simulink model "sampleModel1715"  (R2023a)
settings: Solver=VariableStepAuto  StartTime=0.0  StopTime=10.0  RelTol=1e-3
libraries: hdlsllib x7
settings Model: Creator=user1  LastModifiedBy=user1

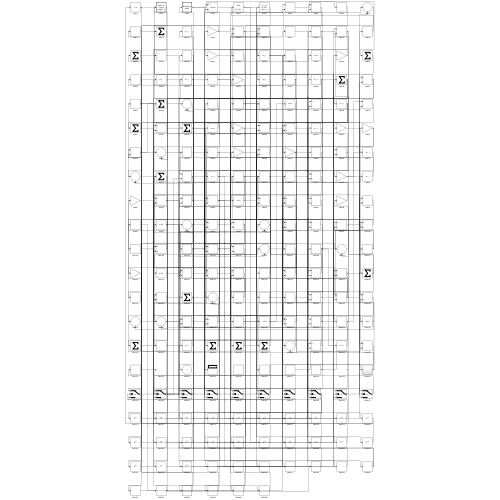
[thumbnail: Simulink's stored preview of the top-level diagram]
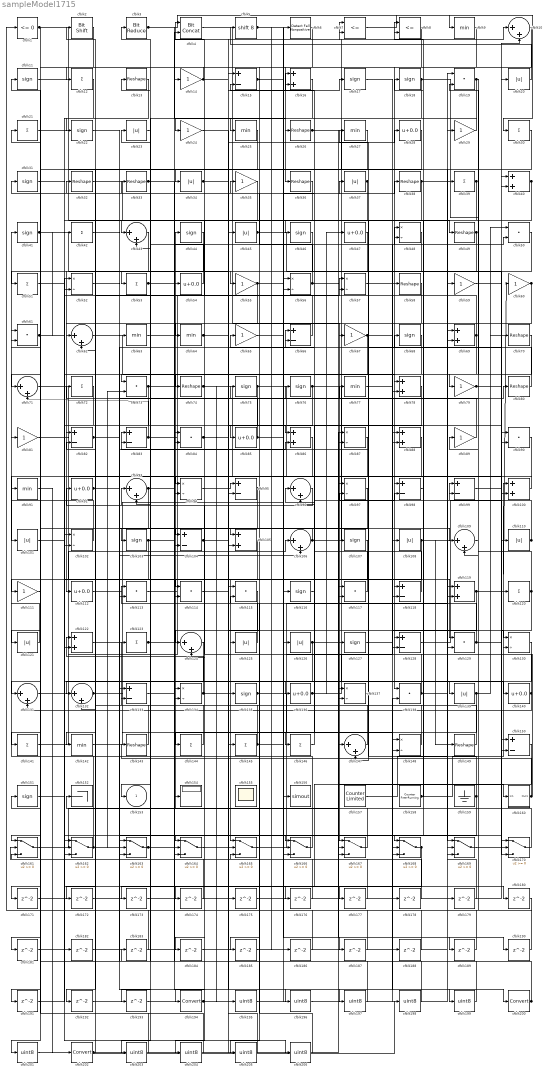
== system sampleModel1715 ==
  cfblk1 : hdlsllib/Logic and Bit Operations/Compare To Zero  relop=<=  OutDataTypeStr=boolean
  cfblk{10,43,62,71,93,96,106,109,124,131..132,147} (12 alike) : Sum  Inputs=|++
  cfblk{16,40,69,78,86,88,100,105,119,122} (10 alike) : Sum
  cfblk{20,23,34,37,45,101,108,110,121,125..126,139} (12 alike) : Abs  SaturateOnIntegerOverflow=off
  cfblk{48,52,56..57,87,94,97,102,130,134,137,148} (12 alike) : Product  Inputs=*/  RndMeth=Zero  SaturateOnIntegerOverflow=on
  cfblk{11,17..18,22,31,41,44,46,68,75..76,103,107,116,127,135,151} (17 alike) : Signum
  cfblk{15,66,82..83,95,98..99,104,118,128,133,150} (12 alike) : Sum  Inputs=+-
  cfblk{14,24,29,35,55,59..60,65,67,79,81,89,111} (13 alike) : Gain
  cfblk{28,47,54,85,92,112,136,140} (8 alike) : Bias  Bias=0.0  SaturateOnIntegerOverflow=off
  cfblk{19,50,61,73,84,90,113..115,117,129,138} (12 alike) : DotProduct  OutDataTypeStr=Inherit: Inherit via internal rule
  cfblk{12,21,30,39,42,51,53,72,120,123,141,144..146} (14 alike) : Sum  Inputs=+
  cfblk{13,26,32..33,36,38,49,58,70,74,80,143,149} (13 alike) : Reshape
  cfblk{9,25,27,63..64,77,91,142} (8 alike) : MinMax
  cfblk152 : Terminator
  cfblk154 : Display
  cfblk155 : Scope
      settings: Floating=on
  cfblk156 : ToWorkspace  VariableName=simout  SaveFormat=Timeseries  SampleTime=-1
  cfblk157 : hdlsllib/Sources/Counter Limited  uplimit=7  tsamp=-1
  cfblk158 : hdlsllib/Sources/Counter Free-Running  NumBits=16  tsamp=-1
  cfblk159 : Ground
  cfblk160 : Subsystem
      settings: LibrarySourceBlock=|
      | hdlsllib/Ports &
      | Subsystems/Subsystem
  cfblk{161..170} (10 alike) : Switch  SaturateOnIntegerOverflow=off  InputSameDT=off
  cfblk{171..193} (23 alike) : Delay  SampleTime=1
  cfblk194 : DataTypeConversion  SaturateOnIntegerOverflow=off  RndMeth=Floor
  cfblk{195..199,201,203..206} (10 alike) : DataTypeConversion  OutDataTypeStr=uint8  SaturateOnIntegerOverflow=off  RndMeth=Floor
  cfblk2 : hdlsllib/Logic and Bit Operations/Bit Shift  mode=Shift Left Logical  N=0
  cfblk200 : DataTypeConversion  SaturateOnIntegerOverflow=off  RndMeth=Floor
  cfblk202 : DataTypeConversion  SaturateOnIntegerOverflow=off  RndMeth=Floor
  cfblk3 : hdlsllib/Logic and Bit Operations/Bit Reduce  mode=AND
  cfblk4 : hdlsllib/Logic and Bit Operations/Bit Concat  numInputs=2
  cfblk5 : ArithShift  BitShiftNumber=8
  cfblk6 : hdlsllib/Logic and Bit Operations/Detect Fall Nonpositive  vinit=0  OutDataTypeStr=boolean
  cfblk7 : RelationalOperator  Operator=<=  OutDataTypeStr=boolean  InputSameDT=off
  cfblk8 : RelationalOperator  Operator=<=  OutDataTypeStr=boolean  InputSameDT=off
  cfblk153 : Outport  VectorParamsAs1DForOutWhenUnconnected=off
  wires:
  cfblk166/1 -> cfblk41/1
  cfblk27/1 -> cfblk34/1
  cfblk11/1 -> cfblk49/1
  cfblk18/1 -> cfblk53/1, cfblk88/2
  cfblk131/1 -> cfblk106/1
  cfblk116/1 -> cfblk65/1
  cfblk127/1 -> cfblk200/1
  cfblk149/1 -> cfblk96/1
  cfblk76/1 -> cfblk139/1, cfblk85/1
  cfblk5/1 -> cfblk186/1, cfblk187/1
  cfblk159/1 -> cfblk83/1, cfblk162/3
  cfblk82/1 -> cfblk66/1, cfblk109/1
  cfblk28/1 -> cfblk141/1
  cfblk143/1 -> cfblk32/1
  cfblk168/1 -> cfblk173/1, cfblk174/1
  cfblk110/1 -> cfblk99/1, cfblk75/1
  cfblk48/1 -> cfblk138/1
  cfblk50/1 -> cfblk112/1
  cfblk162/1 -> cfblk61/1, cfblk84/2, cfblk76/1, cfblk73/2, cfblk166/1, cfblk166/2
  cfblk121/1 -> cfblk81/1
  cfblk55/1 -> cfblk116/1, cfblk95/2
  cfblk4/1 -> cfblk167/1
  cfblk119/1 -> cfblk60/1, cfblk128/2
  cfblk106/1 -> cfblk10/1, cfblk105/1
  cfblk87/1 -> cfblk194/1
  cfblk138/1 -> cfblk59/1, cfblk92/1
  cfblk98/1 -> cfblk168/1
  cfblk167/1 -> cfblk44/1
  cfblk9/1 -> cfblk36/1
  cfblk75/1 -> cfblk168/2, cfblk170/1, cfblk132/2
  cfblk134/1 -> cfblk122/1, cfblk16/2
  cfblk86/1 -> cfblk101/1
  cfblk54/1 -> cfblk23/1
  cfblk165/1 -> cfblk29/1
  cfblk170/1 -> cfblk152/1
  cfblk26/1 -> cfblk88/1, cfblk160/1(In1), cfblk190/1
  cfblk47/1 -> cfblk51/1
  cfblk147/1 -> cfblk54/1
  cfblk141/1 -> cfblk6/1
  cfblk146/1 -> cfblk66/2
  cfblk49/1 -> cfblk104/1, cfblk117/2, cfblk104/2
  cfblk10/1 -> cfblk118/1
  cfblk104/1 -> cfblk15/1, cfblk129/2
  cfblk73/1 -> cfblk154/1, cfblk142/1
  cfblk38/1 -> cfblk64/1, cfblk78/2, cfblk130/1
  cfblk1/1 -> cfblk69/2, cfblk131/1
  cfblk88/1 -> cfblk121/1
  cfblk16/1 -> cfblk43/1
  cfblk107/1 -> cfblk165/1
  cfblk19/1 -> cfblk25/1, cfblk79/1
  cfblk83/1 -> cfblk40/1, cfblk71/2
  cfblk29/1 -> cfblk24/1
  cfblk129/1 -> cfblk20/1, cfblk27/1, cfblk13/1
  cfblk32/1 -> cfblk135/1
  cfblk161/1 -> cfblk107/1
  cfblk60/1 -> cfblk67/1, cfblk147/2
  cfblk15/1 -> cfblk126/1, cfblk185/1
  cfblk52/1 -> cfblk163/1
  cfblk2/1 -> cfblk71/1
  cfblk102/1 -> cfblk21/1
  cfblk128/1 -> cfblk10/2
  cfblk118/1 -> cfblk31/1
  cfblk80/1 -> cfblk57/1
  cfblk78/1 -> cfblk146/1
  cfblk126/1 -> cfblk96/2, cfblk98/2, cfblk164/2
  cfblk122/1 -> cfblk37/1
  cfblk158/1 -> cfblk100/1, cfblk18/1
  cfblk135/1 -> cfblk108/1, cfblk168/3
  cfblk93/1 -> cfblk14/1, cfblk113/2
  cfblk84/1 -> cfblk48/2, cfblk195/1, cfblk199/1
  cfblk13/1 -> cfblk122/2
  cfblk144/1 -> cfblk43/2
  cfblk151/1 -> cfblk57/2
  cfblk62/1 -> cfblk74/1
  cfblk3/1 -> cfblk30/1, cfblk26/1
  cfblk59/1 -> cfblk150/1
  cfblk109/1 -> cfblk19/2
  cfblk163/1 -> cfblk83/2, cfblk86/2
  cfblk113/1 -> cfblk68/1
  cfblk132/1 -> cfblk38/1, cfblk156/1
  cfblk81/1 -> cfblk129/1
  cfblk8/1 -> cfblk55/1
  cfblk21/1 -> cfblk169/1
  cfblk85/1 -> cfblk33/1, cfblk7/2
  cfblk99/1 -> cfblk90/1
  cfblk25/1 -> cfblk62/1
  cfblk43/1 -> cfblk111/1
  cfblk105/1 -> cfblk144/1
  cfblk64/1 -> cfblk86/1, cfblk184/1
  cfblk7/1 -> cfblk9/1
  cfblk42/1 -> cfblk63/1
  cfblk140/1 -> cfblk97/2, cfblk131/2
  cfblk31/1 -> cfblk114/1
  cfblk12/1 -> cfblk22/1
  cfblk164/1 -> cfblk28/1
  cfblk67/1 -> cfblk134/2, cfblk50/2
  cfblk91/1 -> cfblk202/1
  cfblk61/1 -> cfblk140/1, cfblk42/1
  cfblk97/1 -> cfblk161/1
  cfblk103/1 -> cfblk8/2, cfblk48/1, cfblk192/1
  cfblk33/1 -> cfblk103/1, cfblk105/2
  cfblk69/1 -> cfblk4/1, cfblk102/2
  cfblk71/1 -> cfblk100/2
  cfblk89/1 -> cfblk8/1
  cfblk94/1 -> cfblk95/1
  cfblk44/1 -> cfblk73/1
  cfblk123/1 -> cfblk4/2, cfblk193/1
  cfblk157/1 -> cfblk39/1
  cfblk45/1 -> cfblk110/1, cfblk170/2
  cfblk41/1 -> cfblk145/1, cfblk206/1
  cfblk108/1 -> cfblk149/1, cfblk40/2, cfblk191/1
  cfblk14/1 -> cfblk7/1, cfblk12/1
  cfblk46/1 -> cfblk93/2
  cfblk30/1 -> cfblk119/2
  cfblk112/1 -> cfblk56/2
  cfblk56/1 -> cfblk35/1, cfblk118/2, cfblk16/1
  cfblk74/1 -> cfblk98/1, cfblk175/1
  cfblk63/1 -> cfblk114/2
  cfblk100/1 -> cfblk94/1
  cfblk34/1 -> cfblk17/1, cfblk137/1
  cfblk142/1 -> cfblk147/1
  cfblk40/1 -> cfblk125/1, cfblk82/1
  cfblk95/1 -> cfblk124/2, cfblk171/1
  cfblk136/1 -> cfblk58/1, cfblk47/1
  cfblk96/1 -> cfblk94/2
  cfblk79/1 -> cfblk150/2, cfblk70/1
  cfblk90/1 -> cfblk148/2
  cfblk70/1 -> cfblk124/1
  cfblk137/1 -> cfblk77/1
  cfblk58/1 -> cfblk62/2
  cfblk169/1 -> cfblk120/1
  cfblk160/1(Out1) -> cfblk143/1, cfblk130/2
  cfblk120/1 -> cfblk72/1, cfblk89/1, cfblk170/3
  cfblk148/1 -> cfblk3/1
  cfblk23/1 -> cfblk153/1
  cfblk35/1 -> cfblk132/1
  cfblk20/1 -> cfblk5/1
  cfblk125/1 -> cfblk113/1
  cfblk53/1 -> cfblk78/1, cfblk137/2
  cfblk92/1 -> cfblk106/2, cfblk136/1
  cfblk72/1 -> cfblk162/2
  cfblk39/1 -> cfblk117/1, cfblk163/3, cfblk128/1
  cfblk66/1 -> cfblk2/1
  cfblk139/1 -> cfblk164/1, cfblk50/1, cfblk109/2
  cfblk65/1 -> cfblk167/2
  cfblk37/1 -> cfblk52/2, cfblk164/3
  cfblk24/1 -> cfblk46/1
  cfblk117/1 -> cfblk15/2
  cfblk68/1 -> cfblk167/3
  cfblk145/1 -> cfblk123/1, cfblk80/1
  cfblk171/1 -> cfblk163/2
  cfblk124/1 -> cfblk172/1
  cfblk172/1 -> cfblk148/1
  cfblk173/1 -> cfblk19/1
  cfblk174/1 -> cfblk161/2
  cfblk175/1 -> cfblk90/2
  cfblk150/1 -> cfblk176/1
  cfblk176/1 -> cfblk52/1
  cfblk101/1 -> cfblk177/1
  cfblk177/1 -> cfblk134/1
  cfblk57/1 -> cfblk178/1
  cfblk178/1 -> cfblk165/2
  cfblk179/1 -> cfblk69/1
  cfblk114/1 -> cfblk180/1
  cfblk180/1 -> cfblk1/1
  cfblk111/1 -> cfblk181/1
  cfblk181/1 -> cfblk119/1
  cfblk51/1 -> cfblk182/1
  cfblk182/1 -> cfblk169/3
  cfblk183/1 -> cfblk61/2
  cfblk184/1 -> cfblk56/1
  cfblk185/1 -> cfblk165/3
  cfblk186/1 -> cfblk93/1
  cfblk187/1 -> cfblk161/3
  cfblk17/1 -> cfblk188/1
  cfblk188/1 -> cfblk97/1
  cfblk77/1 -> cfblk189/1
  cfblk189/1 -> cfblk162/1
  cfblk190/1 -> cfblk99/2
  cfblk191/1 -> cfblk102/1
  cfblk192/1 -> cfblk169/2
  cfblk193/1 -> cfblk166/3
  cfblk194/1 -> cfblk179/1, cfblk138/2
  cfblk195/1 -> cfblk87/1
  cfblk22/1 -> cfblk196/1
  cfblk196/1 -> cfblk87/2
  cfblk133/1 -> cfblk197/1
  cfblk197/1 -> cfblk183/1
  cfblk198/1 -> cfblk133/1
  cfblk199/1 -> cfblk133/2
  cfblk200/1 -> cfblk84/1, cfblk151/1
  cfblk6/1 -> cfblk201/1
  cfblk201/1 -> cfblk127/1
  cfblk202/1 -> cfblk198/1, cfblk82/2, cfblk45/1
  cfblk36/1 -> cfblk203/1
  cfblk203/1 -> cfblk91/1
  cfblk115/1 -> cfblk204/1
  cfblk204/1 -> cfblk11/1
  cfblk130/1 -> cfblk205/1
  cfblk205/1 -> cfblk115/1
  cfblk206/1 -> cfblk115/2

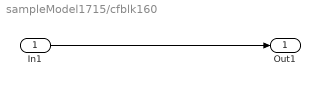
== system sampleModel1715/cfblk160 ==
  In1 : Inport
  Out1 : Outport
  wires:
  In1/1 -> Out1/1
